simulink model "Snowman"  (R2023a)
settings: Solver=FixedStepDiscrete  StartTime=0.0  StopTime=2.0  FixedStep=0.02  RelTol=1e-3
libraries: Rishi_Library x3, simulink x1

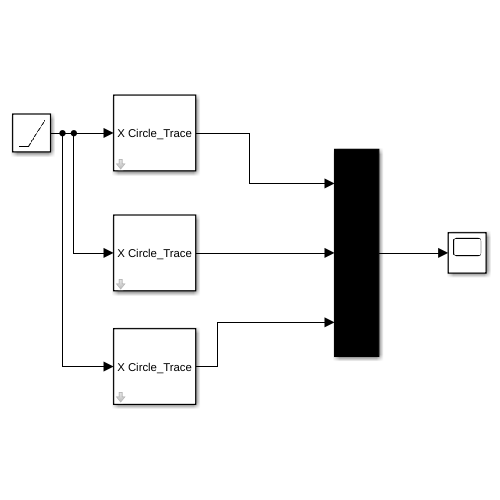
[thumbnail: Simulink's stored preview of the top-level diagram]
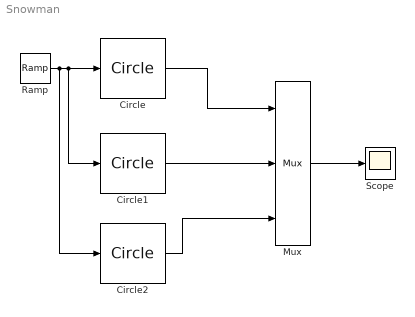
== system Snowman ==
  Circle : Rishi_Library/Circle  X_Offset=0  Y_Offset=0  Radius=0
  Circle1 : Rishi_Library/Circle  X_Offset=0  Y_Offset=2  Radius=1
  Circle2 : Rishi_Library/Circle  X_Offset=0  Y_Offset=4  Radius=2
  Mux : Mux  Inputs=3
  Ramp : simulink/Sources/Ramp  slope=1  start=0  InitialOutput=0
  Scope : Scope
  wires:
  Ramp/1 -> Circle2/1, Circle1/1, Circle/1
  Circle/1 -> Mux/1
  Circle1/1 -> Mux/2
  Circle2/1 -> Mux/3
  Mux/1 -> Scope/1
